simulink model "V_Absorber"  (R2020b)
settings: Solver=VariableStepAuto  StartTime=0.0  StopTime=100  MaxStep=0.001  RelTol=1e-3
PreLoadFcn:
  | M1 = 100
  | M2 = 40
  | b = 50
  | K1 = 50
  | K2 = 50
model workspace (MAT data in the model file):
  K1 = Simulink.Parameter
  K1.Value = 50
  K1.DataType = 'auto'
  K1.Dimensions = [1 1]
  K2 = Simulink.Parameter
  K2.Value = 50
  K2.DataType = 'auto'
  K2.Dimensions = [1 1]
  M1 = Simulink.Parameter
  M1.Value = 100
  M1.DataType = 'auto'
  M1.Dimensions = [1 1]
  M2 = Simulink.Parameter
  M2.Value = 40
  M2.DataType = 'auto'
  M2.Dimensions = [1 1]
  b = Simulink.Parameter
  b.Value = 50
  b.DataType = 'auto'
  b.Dimensions = [1 1]
settings Model: Creator=smart  LastModifiedBy=smart

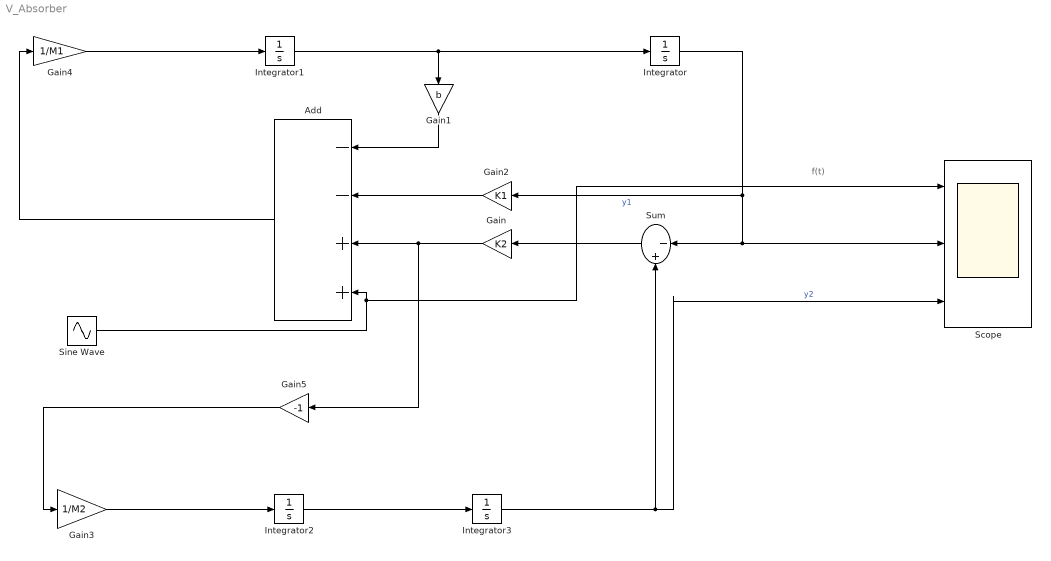
== system V_Absorber ==
  note: f(t)
  Add : Sum  Inputs=--++
  Gain : Gain  Gain=K2
  Gain1 : Gain  Gain=b
  Gain2 : Gain  Gain=K1
  Gain3 : Gain  Gain=1/M2
  Gain4 : Gain  Gain=1/M1
  Gain5 : Gain  Gain=-1
  Integrator{,1..3} (4 alike) : Integrator
  Scope : Scope  NumInputPorts=3
  Sine Wave : Sin  Amplitude=2  Frequency=10  SampleTime=0
  Sum : Sum  Inputs=|-+
  wires:
  Gain2/1 -> Add/2
  Gain/1 -> Gain5/1, Add/3
  Sum/1 -> Gain/1
  Add/1 -> Gain4/1
  Gain4/1 -> Integrator1/1
  Integrator1/1 -> Integrator/1, Gain1/1
  Gain1/1 -> Add/1
  Integrator/1 -> Scope/2, Sum/1, Gain2/1  "y1"
  Integrator2/1 -> Integrator3/1
  Gain3/1 -> Integrator2/1
  Gain5/1 -> Gain3/1
  Integrator3/1 -> Sum/2, Scope/3  "y2"
  Sine Wave/1 -> Scope/1, Add/4
